simulink model "Q2_D"  (R2023b)
settings: Solver=VariableStepAuto  StartTime=0.0  StopTime=20.0  RelTol=1e-3
settings Model: Creator=paria  LastModifiedBy=Amirali

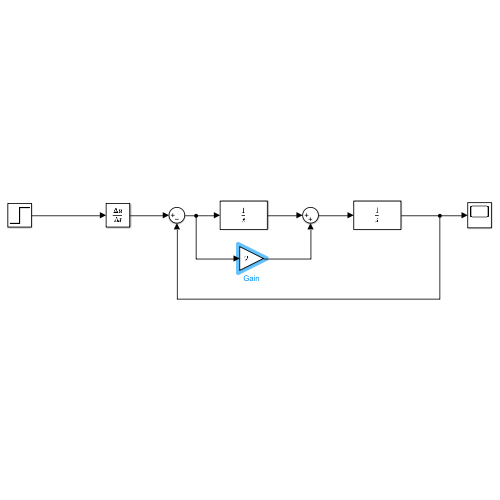
[thumbnail: Simulink's stored preview of the top-level diagram]
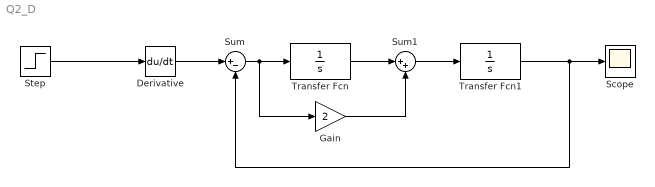
== system Q2_D ==
  Derivative : Derivative
  Gain : Gain  Gain=2
  Scope : Scope
  Step : Step  Time=0.01  SampleTime=0
  Sum : Sum  Inputs=|+-
  Sum1 : Sum  Inputs=|++
  Transfer Fcn : TransferFcn  Denominator=[1 0]
  Transfer Fcn1 : TransferFcn  Denominator=[1 0]
  wires:
  Transfer Fcn1/1 -> Sum/2, Scope/1
  Derivative/1 -> Sum/1
  Transfer Fcn/1 -> Sum1/1
  Gain/1 -> Sum1/2
  Sum/1 -> Gain/1, Transfer Fcn/1
  Step/1 -> Derivative/1
  Sum1/1 -> Transfer Fcn1/1
